simulink model "rr_arm_control"  (R2026a)
settings: Solver=VariableStepAuto  MaxStep=1E-03
InitFcn:
  | rr_arm_control_init;
values from neighbouring files (symbols this model uses):
  b1 = 0.9    [rr_arm_control_init.m]
  b2 = 0.9    [rr_arm_control_init.m]
  g = 9.81    [rr_arm_control_init.m]
  G1 = blkdiag(diag([Ixx1,Iyy1,Izz1]),m1*eye(3))    [rr_arm_control_init.m]
  G2 = blkdiag(diag([Ixx2,Iyy2,Izz2]),m2*eye(3))    [rr_arm_control_init.m]
  M1 = [ ... (first row only)    [rr_arm_control_init.m]
  M2 = [ ... (first row only)    [rr_arm_control_init.m]
  params = [Iyy1,Iyy2,m1,m2,l1,l2,b1,b2,g].'    [rr_arm_control_init.m]
  S1 = rscrew('y',[0,0,0])    [rr_arm_control_init.m]
  S2 = rscrew('y',[l1,0,0])    [rr_arm_control_init.m]
(part 2 of 2)

== system rr_arm_control/gravity_link_2/tform_adjoint/vec2skew ==
  x : Inport
  Constant : Constant  Value=0
  Demux : Demux  Outputs=3
  Gain : Gain  Gain=-1
  Gain1 : Gain  Gain=-1
  Gain2 : Gain  Gain=-1
  Matrix Concatenate : Concatenate  NumInputs=3  Mode=Multidimensional array  ConcatenateDimension=2
  Mux : Mux  Inputs=3
  Mux1 : Mux  Inputs=3
  Mux2 : Mux  Inputs=3
  "[x]" : Outport
  wires:
  Mux1/1 -> Matrix Concatenate/2
  Mux/1 -> Matrix Concatenate/1
  Mux2/1 -> Matrix Concatenate/3
  Matrix Concatenate/1 -> "[x]"/1
  Gain/1 -> Mux/3
  Gain1/1 -> Mux1/1
  Gain2/1 -> Mux2/2
  Constant/1 -> Mux/1, Mux1/2, Mux2/3
  x/1 -> Demux/1
  Demux/3 -> Gain1/1, Mux/2  "z"
  Demux/2 -> Mux2/1, Gain/1  "y"
  Demux/1 -> Gain2/1, Mux1/3  "x"

== system rr_arm_control/link_1/productOfExponentials/Subsystem1 ==
  S : Inport
  q : Inport  Port=2
  Reshape : Reshape  OutputDimensionality=Column vector (2-D)
  Selector : Selector  InputPortWidth=6  IndexOptions=Index vector (dialog)  Indices=1:3  OutputSizes=1
  axisAngleToRotMat : Subsystem
  screwDistanceToPos : Subsystem
  tform : Subsystem
  T : Outport
  wires:
  S/1 -> Reshape/1
  Selector/1 -> axisAngleToRotMat/1(w)  "w"
  q/1 -> screwDistanceToPos/2(q), axisAngleToRotMat/2(q)
  axisAngleToRotMat/1(R) -> tform/1(R)
  tform/1(T) -> T/1
  screwDistanceToPos/1(p) -> tform/2(p)
  Reshape/1 -> screwDistanceToPos/1(S), Selector/1

== system rr_arm_control/link_1/spaceJacobian/angle_screw_to_tform ==
  S : Inport
  q : Inport  Port=2
  Reshape : Reshape  OutputDimensionality=Column vector (2-D)
  Selector : Selector  InputPortWidth=6  IndexOptions=Index vector (dialog)  Indices=1:3  OutputSizes=1
  axisAngleToRotMat : Subsystem
  screwDistanceToPos : Subsystem
  tform : Subsystem
  T : Outport
  wires:
  S/1 -> Reshape/1
  Selector/1 -> axisAngleToRotMat/1(w)  "w"
  q/1 -> screwDistanceToPos/2(q), axisAngleToRotMat/2(q)
  axisAngleToRotMat/1(R) -> tform/1(R)
  tform/1(T) -> T/1
  screwDistanceToPos/1(p) -> tform/2(p)
  Reshape/1 -> screwDistanceToPos/1(S), Selector/1

== system rr_arm_control/link_1/spaceJacobian/tform_adjoint ==
  T : Inport
  Constant : Constant  Value=zeros(3)
  Matrix Concatenate : Concatenate  Mode=Multidimensional array  ConcatenateDimension=2
  Matrix Concatenate1 : Concatenate  Mode=Multidimensional array  ConcatenateDimension=2
  Matrix Concatenate2 : Concatenate  Mode=Multidimensional array
  Matrix Multiply : Product  Multiplication=Matrix(*)
  Selector : Selector  NumberOfDimensions=2  InputPortWidth=3  IndexOptions=Index vector (dialog),Index vector (dialog)  Indices=1:3,1:3  OutputSizes=1,1
  Selector1 : Selector  NumberOfDimensions=2  InputPortWidth=3  IndexOptions=Index vector (dialog),Index vector (dialog)  Indices=1:3,4  OutputSizes=1,1
  vec2skew : Subsystem
  Ad : Outport
  wires:
  Selector1/1 -> vec2skew/1(x)
  Selector/1 -> Matrix Multiply/2, Matrix Concatenate1/2, Matrix Concatenate/1
  Constant/1 -> Matrix Concatenate/2
  vec2skew/1("[x]") -> Matrix Multiply/1
  Matrix Multiply/1 -> Matrix Concatenate1/1
  Matrix Concatenate1/1 -> Matrix Concatenate2/2
  Matrix Concatenate/1 -> Matrix Concatenate2/1
  Matrix Concatenate2/1 -> Ad/1
  T/1 -> Selector1/1, Selector/1

== system rr_arm_control/link_1/spaceJacobianRate/angle_screw_to_tform ==
  S : Inport
  q : Inport  Port=2
  Reshape : Reshape  OutputDimensionality=Column vector (2-D)
  Selector : Selector  InputPortWidth=6  IndexOptions=Index vector (dialog)  Indices=1:3  OutputSizes=1
  axisAngleToRotMat : Subsystem
  screwDistanceToPos : Subsystem
  tform : Subsystem
  T : Outport
  wires:
  S/1 -> Reshape/1
  Selector/1 -> axisAngleToRotMat/1(w)  "w"
  q/1 -> screwDistanceToPos/2(q), axisAngleToRotMat/2(q)
  axisAngleToRotMat/1(R) -> tform/1(R)
  tform/1(T) -> T/1
  screwDistanceToPos/1(p) -> tform/2(p)
  Reshape/1 -> screwDistanceToPos/1(S), Selector/1

== system rr_arm_control/link_1/spaceJacobianRate/tform_adjoint ==
  T : Inport
  Constant : Constant  Value=zeros(3)
  Matrix Concatenate : Concatenate  Mode=Multidimensional array  ConcatenateDimension=2
  Matrix Concatenate1 : Concatenate  Mode=Multidimensional array  ConcatenateDimension=2
  Matrix Concatenate2 : Concatenate  Mode=Multidimensional array
  Matrix Multiply : Product  Multiplication=Matrix(*)
  Selector : Selector  NumberOfDimensions=2  InputPortWidth=3  IndexOptions=Index vector (dialog),Index vector (dialog)  Indices=1:3,1:3  OutputSizes=1,1
  Selector1 : Selector  NumberOfDimensions=2  InputPortWidth=3  IndexOptions=Index vector (dialog),Index vector (dialog)  Indices=1:3,4  OutputSizes=1,1
  vec2skew : Subsystem
  Ad : Outport
  wires:
  Selector1/1 -> vec2skew/1(x)
  Selector/1 -> Matrix Multiply/2, Matrix Concatenate1/2, Matrix Concatenate/1
  Constant/1 -> Matrix Concatenate/2
  vec2skew/1("[x]") -> Matrix Multiply/1
  Matrix Multiply/1 -> Matrix Concatenate1/1
  Matrix Concatenate1/1 -> Matrix Concatenate2/2
  Matrix Concatenate/1 -> Matrix Concatenate2/1
  Matrix Concatenate2/1 -> Ad/1
  T/1 -> Selector1/1, Selector/1

== system rr_arm_control/link_1/spaceJacobianRate/twist_adjoint ==
  V : Inport
  Constant : Constant  Value=zeros(3)
  Matrix Concatenate : Concatenate  Mode=Multidimensional array  ConcatenateDimension=2
  Matrix Concatenate1 : Concatenate  Mode=Multidimensional array  ConcatenateDimension=2
  Matrix Concatenate2 : Concatenate  Mode=Multidimensional array
  Selector : Selector  InputPortWidth=6  IndexOptions=Index vector (dialog)  Indices=1:3  OutputSizes=1
  Selector1 : Selector  InputPortWidth=6  IndexOptions=Index vector (dialog)  Indices=4:6  OutputSizes=1
  "[v]" : Subsystem
  "[w]" : Subsystem
  adV : Outport
  wires:
  Selector/1 -> "[w]"/1(x)
  Constant/1 -> Matrix Concatenate/2
  Matrix Concatenate1/1 -> Matrix Concatenate2/2
  Matrix Concatenate/1 -> Matrix Concatenate2/1
  Matrix Concatenate2/1 -> adV/1
  V/1 -> Selector1/1, Selector/1
  "[w]"/1("[x]") -> Matrix Concatenate1/2, Matrix Concatenate/1
  Selector1/1 -> "[v]"/1(x)
  "[v]"/1("[x]") -> Matrix Concatenate1/1

== system rr_arm_control/link_1/tform_adjoint/vec2skew ==
  x : Inport
  Constant : Constant  Value=0
  Demux : Demux  Outputs=3
  Gain : Gain  Gain=-1
  Gain1 : Gain  Gain=-1
  Gain2 : Gain  Gain=-1
  Matrix Concatenate : Concatenate  NumInputs=3  Mode=Multidimensional array  ConcatenateDimension=2
  Mux : Mux  Inputs=3
  Mux1 : Mux  Inputs=3
  Mux2 : Mux  Inputs=3
  "[x]" : Outport
  wires:
  Mux1/1 -> Matrix Concatenate/2
  Mux/1 -> Matrix Concatenate/1
  Mux2/1 -> Matrix Concatenate/3
  Matrix Concatenate/1 -> "[x]"/1
  Gain/1 -> Mux/3
  Gain1/1 -> Mux1/1
  Gain2/1 -> Mux2/2
  Constant/1 -> Mux/1, Mux1/2, Mux2/3
  x/1 -> Demux/1
  Demux/3 -> Gain1/1, Mux/2  "z"
  Demux/2 -> Mux2/1, Gain/1  "y"
  Demux/1 -> Gain2/1, Mux1/3  "x"

== system rr_arm_control/link_1/twist_adjoint/[v] ==
  x : Inport
  Constant : Constant  Value=0
  Demux : Demux  Outputs=3
  Gain : Gain  Gain=-1
  Gain1 : Gain  Gain=-1
  Gain2 : Gain  Gain=-1
  Matrix Concatenate : Concatenate  NumInputs=3  Mode=Multidimensional array  ConcatenateDimension=2
  Mux : Mux  Inputs=3
  Mux1 : Mux  Inputs=3
  Mux2 : Mux  Inputs=3
  "[x]" : Outport
  wires:
  Mux1/1 -> Matrix Concatenate/2
  Mux/1 -> Matrix Concatenate/1
  Mux2/1 -> Matrix Concatenate/3
  Matrix Concatenate/1 -> "[x]"/1
  Gain/1 -> Mux/3
  Gain1/1 -> Mux1/1
  Gain2/1 -> Mux2/2
  Constant/1 -> Mux/1, Mux1/2, Mux2/3
  x/1 -> Demux/1
  Demux/3 -> Gain1/1, Mux/2  "z"
  Demux/2 -> Mux2/1, Gain/1  "y"
  Demux/1 -> Gain2/1, Mux1/3  "x"

== system rr_arm_control/link_1/twist_adjoint/[w] ==
  x : Inport
  Constant : Constant  Value=0
  Demux : Demux  Outputs=3
  Gain : Gain  Gain=-1
  Gain1 : Gain  Gain=-1
  Gain2 : Gain  Gain=-1
  Matrix Concatenate : Concatenate  NumInputs=3  Mode=Multidimensional array  ConcatenateDimension=2
  Mux : Mux  Inputs=3
  Mux1 : Mux  Inputs=3
  Mux2 : Mux  Inputs=3
  "[x]" : Outport
  wires:
  Mux1/1 -> Matrix Concatenate/2
  Mux/1 -> Matrix Concatenate/1
  Mux2/1 -> Matrix Concatenate/3
  Matrix Concatenate/1 -> "[x]"/1
  Gain/1 -> Mux/3
  Gain1/1 -> Mux1/1
  Gain2/1 -> Mux2/2
  Constant/1 -> Mux/1, Mux1/2, Mux2/3
  x/1 -> Demux/1
  Demux/3 -> Gain1/1, Mux/2  "z"
  Demux/2 -> Mux2/1, Gain/1  "y"
  Demux/1 -> Gain2/1, Mux1/3  "x"

== system rr_arm_control/link_2/productOfExponentials/Subsystem1 ==
  S : Inport
  q : Inport  Port=2
  Reshape : Reshape  OutputDimensionality=Column vector (2-D)
  Selector : Selector  InputPortWidth=6  IndexOptions=Index vector (dialog)  Indices=1:3  OutputSizes=1
  axisAngleToRotMat : Subsystem
  screwDistanceToPos : Subsystem
  tform : Subsystem
  T : Outport
  wires:
  S/1 -> Reshape/1
  Selector/1 -> axisAngleToRotMat/1(w)  "w"
  q/1 -> screwDistanceToPos/2(q), axisAngleToRotMat/2(q)
  axisAngleToRotMat/1(R) -> tform/1(R)
  tform/1(T) -> T/1
  screwDistanceToPos/1(p) -> tform/2(p)
  Reshape/1 -> screwDistanceToPos/1(S), Selector/1

== system rr_arm_control/link_2/spaceJacobian/angle_screw_to_tform ==
  S : Inport
  q : Inport  Port=2
  Reshape : Reshape  OutputDimensionality=Column vector (2-D)
  Selector : Selector  InputPortWidth=6  IndexOptions=Index vector (dialog)  Indices=1:3  OutputSizes=1
  axisAngleToRotMat : Subsystem
  screwDistanceToPos : Subsystem
  tform : Subsystem
  T : Outport
  wires:
  S/1 -> Reshape/1
  Selector/1 -> axisAngleToRotMat/1(w)  "w"
  q/1 -> screwDistanceToPos/2(q), axisAngleToRotMat/2(q)
  axisAngleToRotMat/1(R) -> tform/1(R)
  tform/1(T) -> T/1
  screwDistanceToPos/1(p) -> tform/2(p)
  Reshape/1 -> screwDistanceToPos/1(S), Selector/1

== system rr_arm_control/link_2/spaceJacobian/tform_adjoint ==
  T : Inport
  Constant : Constant  Value=zeros(3)
  Matrix Concatenate : Concatenate  Mode=Multidimensional array  ConcatenateDimension=2
  Matrix Concatenate1 : Concatenate  Mode=Multidimensional array  ConcatenateDimension=2
  Matrix Concatenate2 : Concatenate  Mode=Multidimensional array
  Matrix Multiply : Product  Multiplication=Matrix(*)
  Selector : Selector  NumberOfDimensions=2  InputPortWidth=3  IndexOptions=Index vector (dialog),Index vector (dialog)  Indices=1:3,1:3  OutputSizes=1,1
  Selector1 : Selector  NumberOfDimensions=2  InputPortWidth=3  IndexOptions=Index vector (dialog),Index vector (dialog)  Indices=1:3,4  OutputSizes=1,1
  vec2skew : Subsystem
  Ad : Outport
  wires:
  Selector1/1 -> vec2skew/1(x)
  Selector/1 -> Matrix Multiply/2, Matrix Concatenate1/2, Matrix Concatenate/1
  Constant/1 -> Matrix Concatenate/2
  vec2skew/1("[x]") -> Matrix Multiply/1
  Matrix Multiply/1 -> Matrix Concatenate1/1
  Matrix Concatenate1/1 -> Matrix Concatenate2/2
  Matrix Concatenate/1 -> Matrix Concatenate2/1
  Matrix Concatenate2/1 -> Ad/1
  T/1 -> Selector1/1, Selector/1

== system rr_arm_control/link_2/spaceJacobianRate/angle_screw_to_tform ==
  S : Inport
  q : Inport  Port=2
  Reshape : Reshape  OutputDimensionality=Column vector (2-D)
  Selector : Selector  InputPortWidth=6  IndexOptions=Index vector (dialog)  Indices=1:3  OutputSizes=1
  axisAngleToRotMat : Subsystem
  screwDistanceToPos : Subsystem
  tform : Subsystem
  T : Outport
  wires:
  S/1 -> Reshape/1
  Selector/1 -> axisAngleToRotMat/1(w)  "w"
  q/1 -> screwDistanceToPos/2(q), axisAngleToRotMat/2(q)
  axisAngleToRotMat/1(R) -> tform/1(R)
  tform/1(T) -> T/1
  screwDistanceToPos/1(p) -> tform/2(p)
  Reshape/1 -> screwDistanceToPos/1(S), Selector/1

== system rr_arm_control/link_2/spaceJacobianRate/tform_adjoint ==
  T : Inport
  Constant : Constant  Value=zeros(3)
  Matrix Concatenate : Concatenate  Mode=Multidimensional array  ConcatenateDimension=2
  Matrix Concatenate1 : Concatenate  Mode=Multidimensional array  ConcatenateDimension=2
  Matrix Concatenate2 : Concatenate  Mode=Multidimensional array
  Matrix Multiply : Product  Multiplication=Matrix(*)
  Selector : Selector  NumberOfDimensions=2  InputPortWidth=3  IndexOptions=Index vector (dialog),Index vector (dialog)  Indices=1:3,1:3  OutputSizes=1,1
  Selector1 : Selector  NumberOfDimensions=2  InputPortWidth=3  IndexOptions=Index vector (dialog),Index vector (dialog)  Indices=1:3,4  OutputSizes=1,1
  vec2skew : Subsystem
  Ad : Outport
  wires:
  Selector1/1 -> vec2skew/1(x)
  Selector/1 -> Matrix Multiply/2, Matrix Concatenate1/2, Matrix Concatenate/1
  Constant/1 -> Matrix Concatenate/2
  vec2skew/1("[x]") -> Matrix Multiply/1
  Matrix Multiply/1 -> Matrix Concatenate1/1
  Matrix Concatenate1/1 -> Matrix Concatenate2/2
  Matrix Concatenate/1 -> Matrix Concatenate2/1
  Matrix Concatenate2/1 -> Ad/1
  T/1 -> Selector1/1, Selector/1

== system rr_arm_control/link_2/spaceJacobianRate/twist_adjoint ==
  V : Inport
  Constant : Constant  Value=zeros(3)
  Matrix Concatenate : Concatenate  Mode=Multidimensional array  ConcatenateDimension=2
  Matrix Concatenate1 : Concatenate  Mode=Multidimensional array  ConcatenateDimension=2
  Matrix Concatenate2 : Concatenate  Mode=Multidimensional array
  Selector : Selector  InputPortWidth=6  IndexOptions=Index vector (dialog)  Indices=1:3  OutputSizes=1
  Selector1 : Selector  InputPortWidth=6  IndexOptions=Index vector (dialog)  Indices=4:6  OutputSizes=1
  "[v]" : Subsystem
  "[w]" : Subsystem
  adV : Outport
  wires:
  Selector/1 -> "[w]"/1(x)
  Constant/1 -> Matrix Concatenate/2
  Matrix Concatenate1/1 -> Matrix Concatenate2/2
  Matrix Concatenate/1 -> Matrix Concatenate2/1
  Matrix Concatenate2/1 -> adV/1
  V/1 -> Selector1/1, Selector/1
  "[w]"/1("[x]") -> Matrix Concatenate1/2, Matrix Concatenate/1
  Selector1/1 -> "[v]"/1(x)
  "[v]"/1("[x]") -> Matrix Concatenate1/1

== system rr_arm_control/link_2/tform_adjoint/vec2skew ==
  x : Inport
  Constant : Constant  Value=0
  Demux : Demux  Outputs=3
  Gain : Gain  Gain=-1
  Gain1 : Gain  Gain=-1
  Gain2 : Gain  Gain=-1
  Matrix Concatenate : Concatenate  NumInputs=3  Mode=Multidimensional array  ConcatenateDimension=2
  Mux : Mux  Inputs=3
  Mux1 : Mux  Inputs=3
  Mux2 : Mux  Inputs=3
  "[x]" : Outport
  wires:
  Mux1/1 -> Matrix Concatenate/2
  Mux/1 -> Matrix Concatenate/1
  Mux2/1 -> Matrix Concatenate/3
  Matrix Concatenate/1 -> "[x]"/1
  Gain/1 -> Mux/3
  Gain1/1 -> Mux1/1
  Gain2/1 -> Mux2/2
  Constant/1 -> Mux/1, Mux1/2, Mux2/3
  x/1 -> Demux/1
  Demux/3 -> Gain1/1, Mux/2  "z"
  Demux/2 -> Mux2/1, Gain/1  "y"
  Demux/1 -> Gain2/1, Mux1/3  "x"

== system rr_arm_control/link_2/twist_adjoint/[v] ==
  x : Inport
  Constant : Constant  Value=0
  Demux : Demux  Outputs=3
  Gain : Gain  Gain=-1
  Gain1 : Gain  Gain=-1
  Gain2 : Gain  Gain=-1
  Matrix Concatenate : Concatenate  NumInputs=3  Mode=Multidimensional array  ConcatenateDimension=2
  Mux : Mux  Inputs=3
  Mux1 : Mux  Inputs=3
  Mux2 : Mux  Inputs=3
  "[x]" : Outport
  wires:
  Mux1/1 -> Matrix Concatenate/2
  Mux/1 -> Matrix Concatenate/1
  Mux2/1 -> Matrix Concatenate/3
  Matrix Concatenate/1 -> "[x]"/1
  Gain/1 -> Mux/3
  Gain1/1 -> Mux1/1
  Gain2/1 -> Mux2/2
  Constant/1 -> Mux/1, Mux1/2, Mux2/3
  x/1 -> Demux/1
  Demux/3 -> Gain1/1, Mux/2  "z"
  Demux/2 -> Mux2/1, Gain/1  "y"
  Demux/1 -> Gain2/1, Mux1/3  "x"

== system rr_arm_control/link_2/twist_adjoint/[w] ==
  x : Inport
  Constant : Constant  Value=0
  Demux : Demux  Outputs=3
  Gain : Gain  Gain=-1
  Gain1 : Gain  Gain=-1
  Gain2 : Gain  Gain=-1
  Matrix Concatenate : Concatenate  NumInputs=3  Mode=Multidimensional array  ConcatenateDimension=2
  Mux : Mux  Inputs=3
  Mux1 : Mux  Inputs=3
  Mux2 : Mux  Inputs=3
  "[x]" : Outport
  wires:
  Mux1/1 -> Matrix Concatenate/2
  Mux/1 -> Matrix Concatenate/1
  Mux2/1 -> Matrix Concatenate/3
  Matrix Concatenate/1 -> "[x]"/1
  Gain/1 -> Mux/3
  Gain1/1 -> Mux1/1
  Gain2/1 -> Mux2/2
  Constant/1 -> Mux/1, Mux1/2, Mux2/3
  x/1 -> Demux/1
  Demux/3 -> Gain1/1, Mux/2  "z"
  Demux/2 -> Mux2/1, Gain/1  "y"
  Demux/1 -> Gain2/1, Mux1/3  "x"

== system rr_arm_control/link_1/productOfExponentials/Subsystem1/axisAngleToRotMat ==
  w : Inport
  q : Inport  Port=2
  Constant : Constant
  Cos : Trigonometry  Operator=cos
  I : Constant  Value=eye(3)
  Matrix Multiply : Product  Multiplication=Matrix(*)
  Product : Product
  Product1 : Product
  Sin : Trigonometry
  Sum : Sum  Inputs=|+-
  Sum1 : Sum  Inputs=|++
  Sum2 : Sum  Inputs=|++
  vec2skew : Subsystem
  R : Outport
  wires:
  Cos/1 -> Sum/2
  Sum1/1 -> Sum2/1
  Sum/1 -> Product1/2
  Matrix Multiply/1 -> Product1/1  "[w]^2"
  Product1/1 -> Sum1/2
  Constant/1 -> Sum/1
  Product/1 -> Sum1/1
  I/1 -> Sum2/2
  vec2skew/1("[x]") -> Matrix Multiply/2, Matrix Multiply/1, Product/1  "[w]"
  Sin/1 -> Product/2
  q/1 -> Cos/1, Sin/1
  Sum2/1 -> R/1
  w/1 -> vec2skew/1(x)

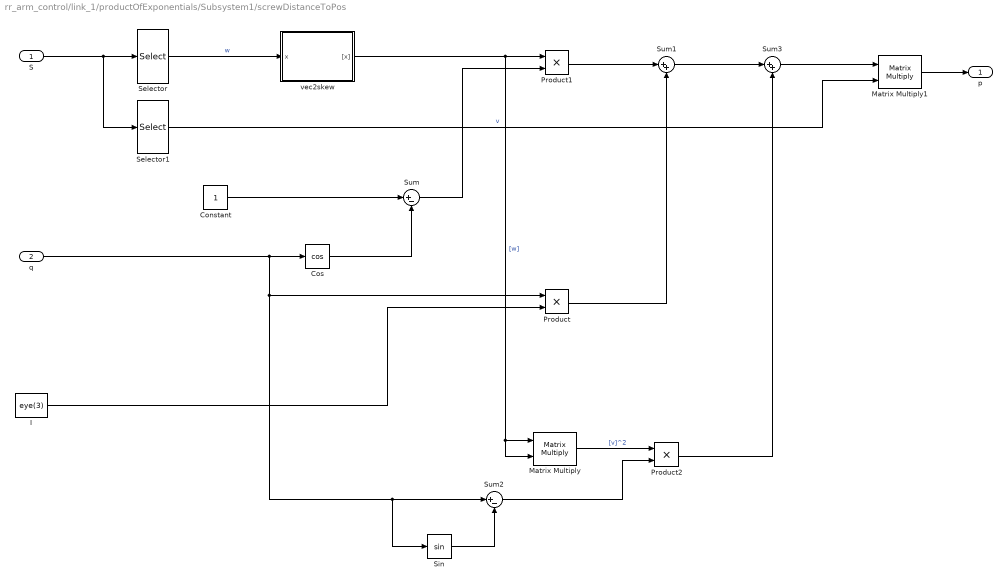
== system rr_arm_control/link_1/productOfExponentials/Subsystem1/screwDistanceToPos ==
  S : Inport
  q : Inport  Port=2
  Constant : Constant
  Cos : Trigonometry  Operator=cos
  I : Constant  Value=eye(3)
  Matrix Multiply : Product  Multiplication=Matrix(*)
  Matrix Multiply1 : Product  Multiplication=Matrix(*)
  Product : Product
  Product1 : Product
  Product2 : Product
  Selector : Selector  InputPortWidth=6  IndexOptions=Index vector (dialog)  Indices=1:3  OutputSizes=1
  Selector1 : Selector  InputPortWidth=6  IndexOptions=Index vector (dialog)  Indices=4:6  OutputSizes=1
  Sin : Trigonometry
  Sum : Sum  Inputs=|+-
  Sum1 : Sum  Inputs=|++
  Sum2 : Sum  Inputs=|+-
  Sum3 : Sum  Inputs=|++
  vec2skew : Subsystem
  p : Outport
  wires:
  Product/1 -> Sum1/2
  q/1 -> Cos/1, Product/1, Sin/1, Sum2/1
  Cos/1 -> Sum/2
  Constant/1 -> Sum/1
  vec2skew/1("[x]") -> Matrix Multiply/2, Matrix Multiply/1, Product1/1  "[w]"
  Sum2/1 -> Product2/2
  I/1 -> Product/2
  Product1/1 -> Sum1/1
  Sum/1 -> Product1/2
  Matrix Multiply/1 -> Product2/1  "[v]^2"
  Sum3/1 -> Matrix Multiply1/1
  Product2/1 -> Sum3/2
  Sin/1 -> Sum2/2
  Sum1/1 -> Sum3/1
  Selector1/1 -> Matrix Multiply1/2  "v"
  Matrix Multiply1/1 -> p/1
  Selector/1 -> vec2skew/1(x)  "w"
  S/1 -> Selector1/1, Selector/1

== system rr_arm_control/link_1/productOfExponentials/Subsystem1/tform ==
  R : Inport
  p : Inport  Port=2
  Constant : Constant  Value=[0,0,0,1]
  Matrix Concatenate : Concatenate  Mode=Multidimensional array  ConcatenateDimension=2
  Matrix Concatenate2 : Concatenate  Mode=Multidimensional array
  Reshape : Reshape  OutputDimensionality=Row vector (2-D)
  T : Outport
  wires:
  p/1 -> Matrix Concatenate/2
  Constant/1 -> Reshape/1
  Matrix Concatenate/1 -> Matrix Concatenate2/1
  Matrix Concatenate2/1 -> T/1
  R/1 -> Matrix Concatenate/1
  Reshape/1 -> Matrix Concatenate2/2

== system rr_arm_control/link_1/spaceJacobian/angle_screw_to_tform/axisAngleToRotMat ==
  w : Inport
  q : Inport  Port=2
  Constant : Constant
  Cos : Trigonometry  Operator=cos
  I : Constant  Value=eye(3)
  Matrix Multiply : Product  Multiplication=Matrix(*)
  Product : Product
  Product1 : Product
  Sin : Trigonometry
  Sum : Sum  Inputs=|+-
  Sum1 : Sum  Inputs=|++
  Sum2 : Sum  Inputs=|++
  vec2skew : Subsystem
  R : Outport
  wires:
  Cos/1 -> Sum/2
  Sum1/1 -> Sum2/1
  Sum/1 -> Product1/2
  Matrix Multiply/1 -> Product1/1  "[w]^2"
  Product1/1 -> Sum1/2
  Constant/1 -> Sum/1
  Product/1 -> Sum1/1
  I/1 -> Sum2/2
  vec2skew/1("[x]") -> Matrix Multiply/2, Matrix Multiply/1, Product/1  "[w]"
  Sin/1 -> Product/2
  q/1 -> Cos/1, Sin/1
  Sum2/1 -> R/1
  w/1 -> vec2skew/1(x)

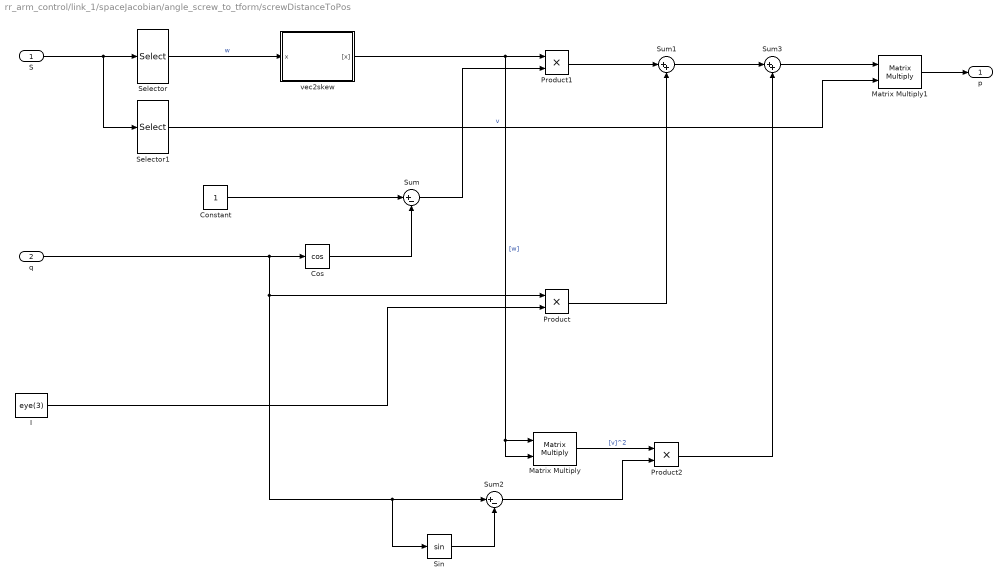
== system rr_arm_control/link_1/spaceJacobian/angle_screw_to_tform/screwDistanceToPos ==
  S : Inport
  q : Inport  Port=2
  Constant : Constant
  Cos : Trigonometry  Operator=cos
  I : Constant  Value=eye(3)
  Matrix Multiply : Product  Multiplication=Matrix(*)
  Matrix Multiply1 : Product  Multiplication=Matrix(*)
  Product : Product
  Product1 : Product
  Product2 : Product
  Selector : Selector  InputPortWidth=6  IndexOptions=Index vector (dialog)  Indices=1:3  OutputSizes=1
  Selector1 : Selector  InputPortWidth=6  IndexOptions=Index vector (dialog)  Indices=4:6  OutputSizes=1
  Sin : Trigonometry
  Sum : Sum  Inputs=|+-
  Sum1 : Sum  Inputs=|++
  Sum2 : Sum  Inputs=|+-
  Sum3 : Sum  Inputs=|++
  vec2skew : Subsystem
  p : Outport
  wires:
  Product/1 -> Sum1/2
  q/1 -> Cos/1, Product/1, Sin/1, Sum2/1
  Cos/1 -> Sum/2
  Constant/1 -> Sum/1
  vec2skew/1("[x]") -> Matrix Multiply/2, Matrix Multiply/1, Product1/1  "[w]"
  Sum2/1 -> Product2/2
  I/1 -> Product/2
  Product1/1 -> Sum1/1
  Sum/1 -> Product1/2
  Matrix Multiply/1 -> Product2/1  "[v]^2"
  Sum3/1 -> Matrix Multiply1/1
  Product2/1 -> Sum3/2
  Sin/1 -> Sum2/2
  Sum1/1 -> Sum3/1
  Selector1/1 -> Matrix Multiply1/2  "v"
  Matrix Multiply1/1 -> p/1
  Selector/1 -> vec2skew/1(x)  "w"
  S/1 -> Selector1/1, Selector/1

== system rr_arm_control/link_1/spaceJacobian/angle_screw_to_tform/tform ==
  R : Inport
  p : Inport  Port=2
  Constant : Constant  Value=[0,0,0,1]
  Matrix Concatenate : Concatenate  Mode=Multidimensional array  ConcatenateDimension=2
  Matrix Concatenate2 : Concatenate  Mode=Multidimensional array
  Reshape : Reshape  OutputDimensionality=Row vector (2-D)
  T : Outport
  wires:
  p/1 -> Matrix Concatenate/2
  Constant/1 -> Reshape/1
  Matrix Concatenate/1 -> Matrix Concatenate2/1
  Matrix Concatenate2/1 -> T/1
  R/1 -> Matrix Concatenate/1
  Reshape/1 -> Matrix Concatenate2/2

== system rr_arm_control/link_1/spaceJacobian/tform_adjoint/vec2skew ==
  x : Inport
  Constant : Constant  Value=0
  Demux : Demux  Outputs=3
  Gain : Gain  Gain=-1
  Gain1 : Gain  Gain=-1
  Gain2 : Gain  Gain=-1
  Matrix Concatenate : Concatenate  NumInputs=3  Mode=Multidimensional array  ConcatenateDimension=2
  Mux : Mux  Inputs=3
  Mux1 : Mux  Inputs=3
  Mux2 : Mux  Inputs=3
  "[x]" : Outport
  wires:
  Mux1/1 -> Matrix Concatenate/2
  Mux/1 -> Matrix Concatenate/1
  Mux2/1 -> Matrix Concatenate/3
  Matrix Concatenate/1 -> "[x]"/1
  Gain/1 -> Mux/3
  Gain1/1 -> Mux1/1
  Gain2/1 -> Mux2/2
  Constant/1 -> Mux/1, Mux1/2, Mux2/3
  x/1 -> Demux/1
  Demux/3 -> Gain1/1, Mux/2  "z"
  Demux/2 -> Mux2/1, Gain/1  "y"
  Demux/1 -> Gain2/1, Mux1/3  "x"

== system rr_arm_control/link_1/spaceJacobianRate/angle_screw_to_tform/axisAngleToRotMat ==
  w : Inport
  q : Inport  Port=2
  Constant : Constant
  Cos : Trigonometry  Operator=cos
  I : Constant  Value=eye(3)
  Matrix Multiply : Product  Multiplication=Matrix(*)
  Product : Product
  Product1 : Product
  Sin : Trigonometry
  Sum : Sum  Inputs=|+-
  Sum1 : Sum  Inputs=|++
  Sum2 : Sum  Inputs=|++
  vec2skew : Subsystem
  R : Outport
  wires:
  Cos/1 -> Sum/2
  Sum1/1 -> Sum2/1
  Sum/1 -> Product1/2
  Matrix Multiply/1 -> Product1/1  "[w]^2"
  Product1/1 -> Sum1/2
  Constant/1 -> Sum/1
  Product/1 -> Sum1/1
  I/1 -> Sum2/2
  vec2skew/1("[x]") -> Matrix Multiply/2, Matrix Multiply/1, Product/1  "[w]"
  Sin/1 -> Product/2
  q/1 -> Cos/1, Sin/1
  Sum2/1 -> R/1
  w/1 -> vec2skew/1(x)

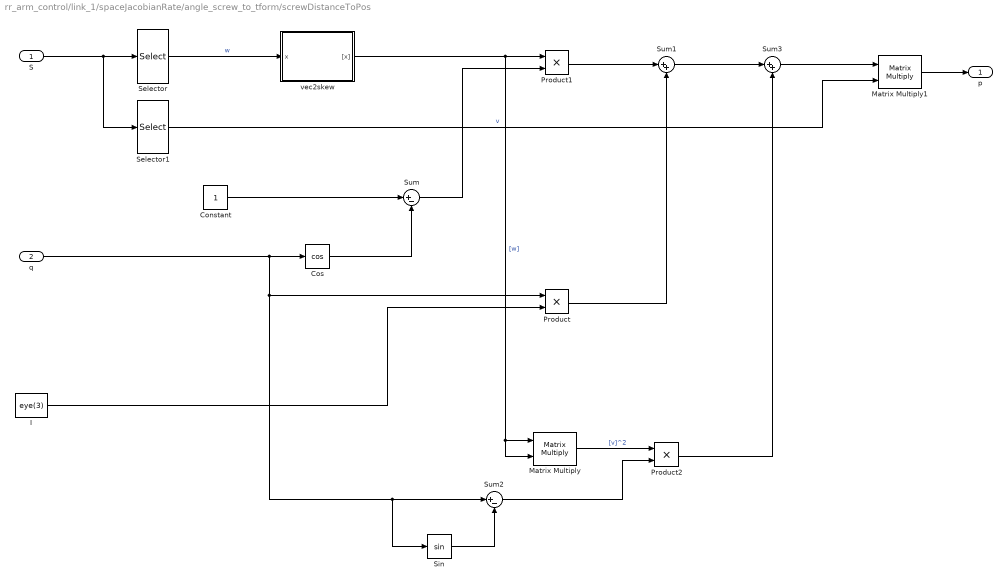
== system rr_arm_control/link_1/spaceJacobianRate/angle_screw_to_tform/screwDistanceToPos ==
  S : Inport
  q : Inport  Port=2
  Constant : Constant
  Cos : Trigonometry  Operator=cos
  I : Constant  Value=eye(3)
  Matrix Multiply : Product  Multiplication=Matrix(*)
  Matrix Multiply1 : Product  Multiplication=Matrix(*)
  Product : Product
  Product1 : Product
  Product2 : Product
  Selector : Selector  InputPortWidth=6  IndexOptions=Index vector (dialog)  Indices=1:3  OutputSizes=1
  Selector1 : Selector  InputPortWidth=6  IndexOptions=Index vector (dialog)  Indices=4:6  OutputSizes=1
  Sin : Trigonometry
  Sum : Sum  Inputs=|+-
  Sum1 : Sum  Inputs=|++
  Sum2 : Sum  Inputs=|+-
  Sum3 : Sum  Inputs=|++
  vec2skew : Subsystem
  p : Outport
  wires:
  Product/1 -> Sum1/2
  q/1 -> Cos/1, Product/1, Sin/1, Sum2/1
  Cos/1 -> Sum/2
  Constant/1 -> Sum/1
  vec2skew/1("[x]") -> Matrix Multiply/2, Matrix Multiply/1, Product1/1  "[w]"
  Sum2/1 -> Product2/2
  I/1 -> Product/2
  Product1/1 -> Sum1/1
  Sum/1 -> Product1/2
  Matrix Multiply/1 -> Product2/1  "[v]^2"
  Sum3/1 -> Matrix Multiply1/1
  Product2/1 -> Sum3/2
  Sin/1 -> Sum2/2
  Sum1/1 -> Sum3/1
  Selector1/1 -> Matrix Multiply1/2  "v"
  Matrix Multiply1/1 -> p/1
  Selector/1 -> vec2skew/1(x)  "w"
  S/1 -> Selector1/1, Selector/1

== system rr_arm_control/link_1/spaceJacobianRate/angle_screw_to_tform/tform ==
  R : Inport
  p : Inport  Port=2
  Constant : Constant  Value=[0,0,0,1]
  Matrix Concatenate : Concatenate  Mode=Multidimensional array  ConcatenateDimension=2
  Matrix Concatenate2 : Concatenate  Mode=Multidimensional array
  Reshape : Reshape  OutputDimensionality=Row vector (2-D)
  T : Outport
  wires:
  p/1 -> Matrix Concatenate/2
  Constant/1 -> Reshape/1
  Matrix Concatenate/1 -> Matrix Concatenate2/1
  Matrix Concatenate2/1 -> T/1
  R/1 -> Matrix Concatenate/1
  Reshape/1 -> Matrix Concatenate2/2

== system rr_arm_control/link_1/spaceJacobianRate/tform_adjoint/vec2skew ==
  x : Inport
  Constant : Constant  Value=0
  Demux : Demux  Outputs=3
  Gain : Gain  Gain=-1
  Gain1 : Gain  Gain=-1
  Gain2 : Gain  Gain=-1
  Matrix Concatenate : Concatenate  NumInputs=3  Mode=Multidimensional array  ConcatenateDimension=2
  Mux : Mux  Inputs=3
  Mux1 : Mux  Inputs=3
  Mux2 : Mux  Inputs=3
  "[x]" : Outport
  wires:
  Mux1/1 -> Matrix Concatenate/2
  Mux/1 -> Matrix Concatenate/1
  Mux2/1 -> Matrix Concatenate/3
  Matrix Concatenate/1 -> "[x]"/1
  Gain/1 -> Mux/3
  Gain1/1 -> Mux1/1
  Gain2/1 -> Mux2/2
  Constant/1 -> Mux/1, Mux1/2, Mux2/3
  x/1 -> Demux/1
  Demux/3 -> Gain1/1, Mux/2  "z"
  Demux/2 -> Mux2/1, Gain/1  "y"
  Demux/1 -> Gain2/1, Mux1/3  "x"

== system rr_arm_control/link_1/spaceJacobianRate/twist_adjoint/[v] ==
  x : Inport
  Constant : Constant  Value=0
  Demux : Demux  Outputs=3
  Gain : Gain  Gain=-1
  Gain1 : Gain  Gain=-1
  Gain2 : Gain  Gain=-1
  Matrix Concatenate : Concatenate  NumInputs=3  Mode=Multidimensional array  ConcatenateDimension=2
  Mux : Mux  Inputs=3
  Mux1 : Mux  Inputs=3
  Mux2 : Mux  Inputs=3
  "[x]" : Outport
  wires:
  Mux1/1 -> Matrix Concatenate/2
  Mux/1 -> Matrix Concatenate/1
  Mux2/1 -> Matrix Concatenate/3
  Matrix Concatenate/1 -> "[x]"/1
  Gain/1 -> Mux/3
  Gain1/1 -> Mux1/1
  Gain2/1 -> Mux2/2
  Constant/1 -> Mux/1, Mux1/2, Mux2/3
  x/1 -> Demux/1
  Demux/3 -> Gain1/1, Mux/2  "z"
  Demux/2 -> Mux2/1, Gain/1  "y"
  Demux/1 -> Gain2/1, Mux1/3  "x"

== system rr_arm_control/link_1/spaceJacobianRate/twist_adjoint/[w] ==
  x : Inport
  Constant : Constant  Value=0
  Demux : Demux  Outputs=3
  Gain : Gain  Gain=-1
  Gain1 : Gain  Gain=-1
  Gain2 : Gain  Gain=-1
  Matrix Concatenate : Concatenate  NumInputs=3  Mode=Multidimensional array  ConcatenateDimension=2
  Mux : Mux  Inputs=3
  Mux1 : Mux  Inputs=3
  Mux2 : Mux  Inputs=3
  "[x]" : Outport
  wires:
  Mux1/1 -> Matrix Concatenate/2
  Mux/1 -> Matrix Concatenate/1
  Mux2/1 -> Matrix Concatenate/3
  Matrix Concatenate/1 -> "[x]"/1
  Gain/1 -> Mux/3
  Gain1/1 -> Mux1/1
  Gain2/1 -> Mux2/2
  Constant/1 -> Mux/1, Mux1/2, Mux2/3
  x/1 -> Demux/1
  Demux/3 -> Gain1/1, Mux/2  "z"
  Demux/2 -> Mux2/1, Gain/1  "y"
  Demux/1 -> Gain2/1, Mux1/3  "x"

== system rr_arm_control/link_2/productOfExponentials/Subsystem1/axisAngleToRotMat ==
  w : Inport
  q : Inport  Port=2
  Constant : Constant
  Cos : Trigonometry  Operator=cos
  I : Constant  Value=eye(3)
  Matrix Multiply : Product  Multiplication=Matrix(*)
  Product : Product
  Product1 : Product
  Sin : Trigonometry
  Sum : Sum  Inputs=|+-
  Sum1 : Sum  Inputs=|++
  Sum2 : Sum  Inputs=|++
  vec2skew : Subsystem
  R : Outport
  wires:
  Cos/1 -> Sum/2
  Sum1/1 -> Sum2/1
  Sum/1 -> Product1/2
  Matrix Multiply/1 -> Product1/1  "[w]^2"
  Product1/1 -> Sum1/2
  Constant/1 -> Sum/1
  Product/1 -> Sum1/1
  I/1 -> Sum2/2
  vec2skew/1("[x]") -> Matrix Multiply/2, Matrix Multiply/1, Product/1  "[w]"
  Sin/1 -> Product/2
  q/1 -> Cos/1, Sin/1
  Sum2/1 -> R/1
  w/1 -> vec2skew/1(x)

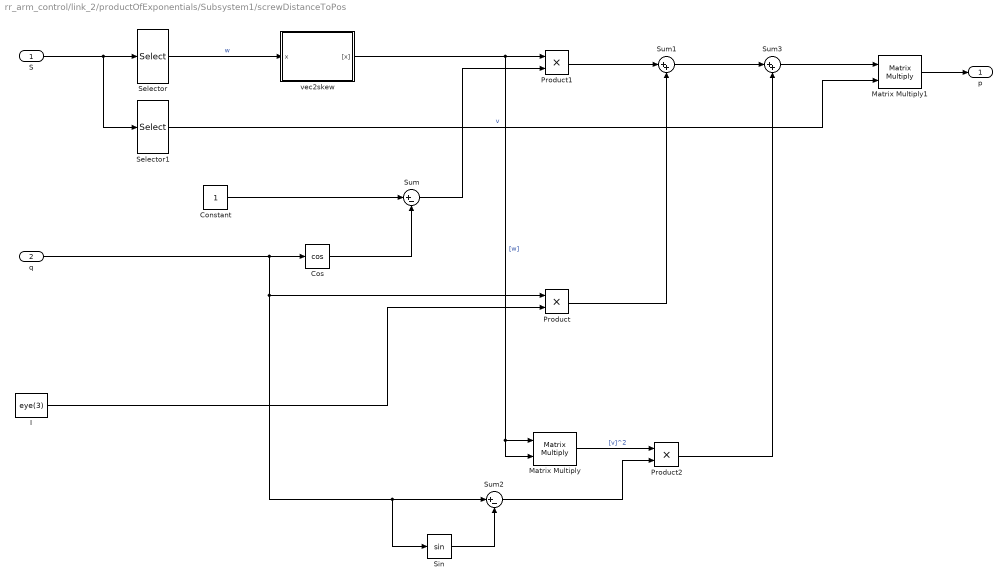
== system rr_arm_control/link_2/productOfExponentials/Subsystem1/screwDistanceToPos ==
  S : Inport
  q : Inport  Port=2
  Constant : Constant
  Cos : Trigonometry  Operator=cos
  I : Constant  Value=eye(3)
  Matrix Multiply : Product  Multiplication=Matrix(*)
  Matrix Multiply1 : Product  Multiplication=Matrix(*)
  Product : Product
  Product1 : Product
  Product2 : Product
  Selector : Selector  InputPortWidth=6  IndexOptions=Index vector (dialog)  Indices=1:3  OutputSizes=1
  Selector1 : Selector  InputPortWidth=6  IndexOptions=Index vector (dialog)  Indices=4:6  OutputSizes=1
  Sin : Trigonometry
  Sum : Sum  Inputs=|+-
  Sum1 : Sum  Inputs=|++
  Sum2 : Sum  Inputs=|+-
  Sum3 : Sum  Inputs=|++
  vec2skew : Subsystem
  p : Outport
  wires:
  Product/1 -> Sum1/2
  q/1 -> Cos/1, Product/1, Sin/1, Sum2/1
  Cos/1 -> Sum/2
  Constant/1 -> Sum/1
  vec2skew/1("[x]") -> Matrix Multiply/2, Matrix Multiply/1, Product1/1  "[w]"
  Sum2/1 -> Product2/2
  I/1 -> Product/2
  Product1/1 -> Sum1/1
  Sum/1 -> Product1/2
  Matrix Multiply/1 -> Product2/1  "[v]^2"
  Sum3/1 -> Matrix Multiply1/1
  Product2/1 -> Sum3/2
  Sin/1 -> Sum2/2
  Sum1/1 -> Sum3/1
  Selector1/1 -> Matrix Multiply1/2  "v"
  Matrix Multiply1/1 -> p/1
  Selector/1 -> vec2skew/1(x)  "w"
  S/1 -> Selector1/1, Selector/1

== system rr_arm_control/link_2/productOfExponentials/Subsystem1/tform ==
  R : Inport
  p : Inport  Port=2
  Constant : Constant  Value=[0,0,0,1]
  Matrix Concatenate : Concatenate  Mode=Multidimensional array  ConcatenateDimension=2
  Matrix Concatenate2 : Concatenate  Mode=Multidimensional array
  Reshape : Reshape  OutputDimensionality=Row vector (2-D)
  T : Outport
  wires:
  p/1 -> Matrix Concatenate/2
  Constant/1 -> Reshape/1
  Matrix Concatenate/1 -> Matrix Concatenate2/1
  Matrix Concatenate2/1 -> T/1
  R/1 -> Matrix Concatenate/1
  Reshape/1 -> Matrix Concatenate2/2

== system rr_arm_control/link_2/spaceJacobian/angle_screw_to_tform/axisAngleToRotMat ==
  w : Inport
  q : Inport  Port=2
  Constant : Constant
  Cos : Trigonometry  Operator=cos
  I : Constant  Value=eye(3)
  Matrix Multiply : Product  Multiplication=Matrix(*)
  Product : Product
  Product1 : Product
  Sin : Trigonometry
  Sum : Sum  Inputs=|+-
  Sum1 : Sum  Inputs=|++
  Sum2 : Sum  Inputs=|++
  vec2skew : Subsystem
  R : Outport
  wires:
  Cos/1 -> Sum/2
  Sum1/1 -> Sum2/1
  Sum/1 -> Product1/2
  Matrix Multiply/1 -> Product1/1  "[w]^2"
  Product1/1 -> Sum1/2
  Constant/1 -> Sum/1
  Product/1 -> Sum1/1
  I/1 -> Sum2/2
  vec2skew/1("[x]") -> Matrix Multiply/2, Matrix Multiply/1, Product/1  "[w]"
  Sin/1 -> Product/2
  q/1 -> Cos/1, Sin/1
  Sum2/1 -> R/1
  w/1 -> vec2skew/1(x)

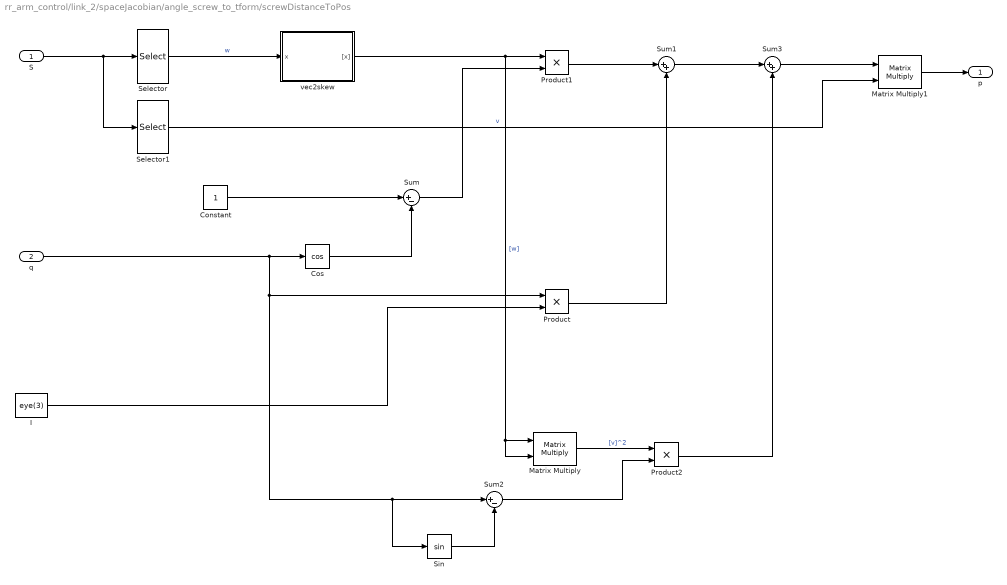
== system rr_arm_control/link_2/spaceJacobian/angle_screw_to_tform/screwDistanceToPos ==
  S : Inport
  q : Inport  Port=2
  Constant : Constant
  Cos : Trigonometry  Operator=cos
  I : Constant  Value=eye(3)
  Matrix Multiply : Product  Multiplication=Matrix(*)
  Matrix Multiply1 : Product  Multiplication=Matrix(*)
  Product : Product
  Product1 : Product
  Product2 : Product
  Selector : Selector  InputPortWidth=6  IndexOptions=Index vector (dialog)  Indices=1:3  OutputSizes=1
  Selector1 : Selector  InputPortWidth=6  IndexOptions=Index vector (dialog)  Indices=4:6  OutputSizes=1
  Sin : Trigonometry
  Sum : Sum  Inputs=|+-
  Sum1 : Sum  Inputs=|++
  Sum2 : Sum  Inputs=|+-
  Sum3 : Sum  Inputs=|++
  vec2skew : Subsystem
  p : Outport
  wires:
  Product/1 -> Sum1/2
  q/1 -> Cos/1, Product/1, Sin/1, Sum2/1
  Cos/1 -> Sum/2
  Constant/1 -> Sum/1
  vec2skew/1("[x]") -> Matrix Multiply/2, Matrix Multiply/1, Product1/1  "[w]"
  Sum2/1 -> Product2/2
  I/1 -> Product/2
  Product1/1 -> Sum1/1
  Sum/1 -> Product1/2
  Matrix Multiply/1 -> Product2/1  "[v]^2"
  Sum3/1 -> Matrix Multiply1/1
  Product2/1 -> Sum3/2
  Sin/1 -> Sum2/2
  Sum1/1 -> Sum3/1
  Selector1/1 -> Matrix Multiply1/2  "v"
  Matrix Multiply1/1 -> p/1
  Selector/1 -> vec2skew/1(x)  "w"
  S/1 -> Selector1/1, Selector/1

== system rr_arm_control/link_2/spaceJacobian/angle_screw_to_tform/tform ==
  R : Inport
  p : Inport  Port=2
  Constant : Constant  Value=[0,0,0,1]
  Matrix Concatenate : Concatenate  Mode=Multidimensional array  ConcatenateDimension=2
  Matrix Concatenate2 : Concatenate  Mode=Multidimensional array
  Reshape : Reshape  OutputDimensionality=Row vector (2-D)
  T : Outport
  wires:
  p/1 -> Matrix Concatenate/2
  Constant/1 -> Reshape/1
  Matrix Concatenate/1 -> Matrix Concatenate2/1
  Matrix Concatenate2/1 -> T/1
  R/1 -> Matrix Concatenate/1
  Reshape/1 -> Matrix Concatenate2/2

== system rr_arm_control/link_2/spaceJacobian/tform_adjoint/vec2skew ==
  x : Inport
  Constant : Constant  Value=0
  Demux : Demux  Outputs=3
  Gain : Gain  Gain=-1
  Gain1 : Gain  Gain=-1
  Gain2 : Gain  Gain=-1
  Matrix Concatenate : Concatenate  NumInputs=3  Mode=Multidimensional array  ConcatenateDimension=2
  Mux : Mux  Inputs=3
  Mux1 : Mux  Inputs=3
  Mux2 : Mux  Inputs=3
  "[x]" : Outport
  wires:
  Mux1/1 -> Matrix Concatenate/2
  Mux/1 -> Matrix Concatenate/1
  Mux2/1 -> Matrix Concatenate/3
  Matrix Concatenate/1 -> "[x]"/1
  Gain/1 -> Mux/3
  Gain1/1 -> Mux1/1
  Gain2/1 -> Mux2/2
  Constant/1 -> Mux/1, Mux1/2, Mux2/3
  x/1 -> Demux/1
  Demux/3 -> Gain1/1, Mux/2  "z"
  Demux/2 -> Mux2/1, Gain/1  "y"
  Demux/1 -> Gain2/1, Mux1/3  "x"

== system rr_arm_control/link_2/spaceJacobianRate/angle_screw_to_tform/axisAngleToRotMat ==
  w : Inport
  q : Inport  Port=2
  Constant : Constant
  Cos : Trigonometry  Operator=cos
  I : Constant  Value=eye(3)
  Matrix Multiply : Product  Multiplication=Matrix(*)
  Product : Product
  Product1 : Product
  Sin : Trigonometry
  Sum : Sum  Inputs=|+-
  Sum1 : Sum  Inputs=|++
  Sum2 : Sum  Inputs=|++
  vec2skew : Subsystem
  R : Outport
  wires:
  Cos/1 -> Sum/2
  Sum1/1 -> Sum2/1
  Sum/1 -> Product1/2
  Matrix Multiply/1 -> Product1/1  "[w]^2"
  Product1/1 -> Sum1/2
  Constant/1 -> Sum/1
  Product/1 -> Sum1/1
  I/1 -> Sum2/2
  vec2skew/1("[x]") -> Matrix Multiply/2, Matrix Multiply/1, Product/1  "[w]"
  Sin/1 -> Product/2
  q/1 -> Cos/1, Sin/1
  Sum2/1 -> R/1
  w/1 -> vec2skew/1(x)

== system rr_arm_control/link_2/spaceJacobianRate/angle_screw_to_tform/screwDistanceToPos ==
  S : Inport
  q : Inport  Port=2
  Constant : Constant
  Cos : Trigonometry  Operator=cos
  I : Constant  Value=eye(3)
  Matrix Multiply : Product  Multiplication=Matrix(*)
  Matrix Multiply1 : Product  Multiplication=Matrix(*)
  Product : Product
  Product1 : Product
  Product2 : Product
  Selector : Selector  InputPortWidth=6  IndexOptions=Index vector (dialog)  Indices=1:3  OutputSizes=1
  Selector1 : Selector  InputPortWidth=6  IndexOptions=Index vector (dialog)  Indices=4:6  OutputSizes=1
  Sin : Trigonometry
  Sum : Sum  Inputs=|+-
  Sum1 : Sum  Inputs=|++
  Sum2 : Sum  Inputs=|+-
  Sum3 : Sum  Inputs=|++
  vec2skew : Subsystem
  p : Outport
  wires:
  Product/1 -> Sum1/2
  q/1 -> Cos/1, Product/1, Sin/1, Sum2/1
  Cos/1 -> Sum/2
  Constant/1 -> Sum/1
  vec2skew/1("[x]") -> Matrix Multiply/2, Matrix Multiply/1, Product1/1  "[w]"
  Sum2/1 -> Product2/2
  I/1 -> Product/2
  Product1/1 -> Sum1/1
  Sum/1 -> Product1/2
  Matrix Multiply/1 -> Product2/1  "[v]^2"
  Sum3/1 -> Matrix Multiply1/1
  Product2/1 -> Sum3/2
  Sin/1 -> Sum2/2
  Sum1/1 -> Sum3/1
  Selector1/1 -> Matrix Multiply1/2  "v"
  Matrix Multiply1/1 -> p/1
  Selector/1 -> vec2skew/1(x)  "w"
  S/1 -> Selector1/1, Selector/1

== system rr_arm_control/link_2/spaceJacobianRate/angle_screw_to_tform/tform ==
  R : Inport
  p : Inport  Port=2
  Constant : Constant  Value=[0,0,0,1]
  Matrix Concatenate : Concatenate  Mode=Multidimensional array  ConcatenateDimension=2
  Matrix Concatenate2 : Concatenate  Mode=Multidimensional array
  Reshape : Reshape  OutputDimensionality=Row vector (2-D)
  T : Outport
  wires:
  p/1 -> Matrix Concatenate/2
  Constant/1 -> Reshape/1
  Matrix Concatenate/1 -> Matrix Concatenate2/1
  Matrix Concatenate2/1 -> T/1
  R/1 -> Matrix Concatenate/1
  Reshape/1 -> Matrix Concatenate2/2

== system rr_arm_control/link_2/spaceJacobianRate/tform_adjoint/vec2skew ==
  x : Inport
  Constant : Constant  Value=0
  Demux : Demux  Outputs=3
  Gain : Gain  Gain=-1
  Gain1 : Gain  Gain=-1
  Gain2 : Gain  Gain=-1
  Matrix Concatenate : Concatenate  NumInputs=3  Mode=Multidimensional array  ConcatenateDimension=2
  Mux : Mux  Inputs=3
  Mux1 : Mux  Inputs=3
  Mux2 : Mux  Inputs=3
  "[x]" : Outport
  wires:
  Mux1/1 -> Matrix Concatenate/2
  Mux/1 -> Matrix Concatenate/1
  Mux2/1 -> Matrix Concatenate/3
  Matrix Concatenate/1 -> "[x]"/1
  Gain/1 -> Mux/3
  Gain1/1 -> Mux1/1
  Gain2/1 -> Mux2/2
  Constant/1 -> Mux/1, Mux1/2, Mux2/3
  x/1 -> Demux/1
  Demux/3 -> Gain1/1, Mux/2  "z"
  Demux/2 -> Mux2/1, Gain/1  "y"
  Demux/1 -> Gain2/1, Mux1/3  "x"

== system rr_arm_control/link_2/spaceJacobianRate/twist_adjoint/[v] ==
  x : Inport
  Constant : Constant  Value=0
  Demux : Demux  Outputs=3
  Gain : Gain  Gain=-1
  Gain1 : Gain  Gain=-1
  Gain2 : Gain  Gain=-1
  Matrix Concatenate : Concatenate  NumInputs=3  Mode=Multidimensional array  ConcatenateDimension=2
  Mux : Mux  Inputs=3
  Mux1 : Mux  Inputs=3
  Mux2 : Mux  Inputs=3
  "[x]" : Outport
  wires:
  Mux1/1 -> Matrix Concatenate/2
  Mux/1 -> Matrix Concatenate/1
  Mux2/1 -> Matrix Concatenate/3
  Matrix Concatenate/1 -> "[x]"/1
  Gain/1 -> Mux/3
  Gain1/1 -> Mux1/1
  Gain2/1 -> Mux2/2
  Constant/1 -> Mux/1, Mux1/2, Mux2/3
  x/1 -> Demux/1
  Demux/3 -> Gain1/1, Mux/2  "z"
  Demux/2 -> Mux2/1, Gain/1  "y"
  Demux/1 -> Gain2/1, Mux1/3  "x"

== system rr_arm_control/link_2/spaceJacobianRate/twist_adjoint/[w] ==
  x : Inport
  Constant : Constant  Value=0
  Demux : Demux  Outputs=3
  Gain : Gain  Gain=-1
  Gain1 : Gain  Gain=-1
  Gain2 : Gain  Gain=-1
  Matrix Concatenate : Concatenate  NumInputs=3  Mode=Multidimensional array  ConcatenateDimension=2
  Mux : Mux  Inputs=3
  Mux1 : Mux  Inputs=3
  Mux2 : Mux  Inputs=3
  "[x]" : Outport
  wires:
  Mux1/1 -> Matrix Concatenate/2
  Mux/1 -> Matrix Concatenate/1
  Mux2/1 -> Matrix Concatenate/3
  Matrix Concatenate/1 -> "[x]"/1
  Gain/1 -> Mux/3
  Gain1/1 -> Mux1/1
  Gain2/1 -> Mux2/2
  Constant/1 -> Mux/1, Mux1/2, Mux2/3
  x/1 -> Demux/1
  Demux/3 -> Gain1/1, Mux/2  "z"
  Demux/2 -> Mux2/1, Gain/1  "y"
  Demux/1 -> Gain2/1, Mux1/3  "x"

== system rr_arm_control/link_1/productOfExponentials/Subsystem1/axisAngleToRotMat/vec2skew ==
  x : Inport
  Constant : Constant  Value=0
  Demux : Demux  Outputs=3
  Gain : Gain  Gain=-1
  Gain1 : Gain  Gain=-1
  Gain2 : Gain  Gain=-1
  Matrix Concatenate : Concatenate  NumInputs=3  Mode=Multidimensional array  ConcatenateDimension=2
  Mux : Mux  Inputs=3
  Mux1 : Mux  Inputs=3
  Mux2 : Mux  Inputs=3
  "[x]" : Outport
  wires:
  Mux1/1 -> Matrix Concatenate/2
  Mux/1 -> Matrix Concatenate/1
  Mux2/1 -> Matrix Concatenate/3
  Matrix Concatenate/1 -> "[x]"/1
  Gain/1 -> Mux/3
  Gain1/1 -> Mux1/1
  Gain2/1 -> Mux2/2
  Constant/1 -> Mux/1, Mux1/2, Mux2/3
  x/1 -> Demux/1
  Demux/3 -> Gain1/1, Mux/2  "z"
  Demux/2 -> Mux2/1, Gain/1  "y"
  Demux/1 -> Gain2/1, Mux1/3  "x"

== system rr_arm_control/link_1/productOfExponentials/Subsystem1/screwDistanceToPos/vec2skew ==
  x : Inport
  Constant : Constant  Value=0
  Demux : Demux  Outputs=3
  Gain : Gain  Gain=-1
  Gain1 : Gain  Gain=-1
  Gain2 : Gain  Gain=-1
  Matrix Concatenate : Concatenate  NumInputs=3  Mode=Multidimensional array  ConcatenateDimension=2
  Mux : Mux  Inputs=3
  Mux1 : Mux  Inputs=3
  Mux2 : Mux  Inputs=3
  "[x]" : Outport
  wires:
  Mux1/1 -> Matrix Concatenate/2
  Mux/1 -> Matrix Concatenate/1
  Mux2/1 -> Matrix Concatenate/3
  Matrix Concatenate/1 -> "[x]"/1
  Gain/1 -> Mux/3
  Gain1/1 -> Mux1/1
  Gain2/1 -> Mux2/2
  Constant/1 -> Mux/1, Mux1/2, Mux2/3
  x/1 -> Demux/1
  Demux/3 -> Gain1/1, Mux/2  "z"
  Demux/2 -> Mux2/1, Gain/1  "y"
  Demux/1 -> Gain2/1, Mux1/3  "x"

== system rr_arm_control/link_1/spaceJacobian/angle_screw_to_tform/axisAngleToRotMat/vec2skew ==
  x : Inport
  Constant : Constant  Value=0
  Demux : Demux  Outputs=3
  Gain : Gain  Gain=-1
  Gain1 : Gain  Gain=-1
  Gain2 : Gain  Gain=-1
  Matrix Concatenate : Concatenate  NumInputs=3  Mode=Multidimensional array  ConcatenateDimension=2
  Mux : Mux  Inputs=3
  Mux1 : Mux  Inputs=3
  Mux2 : Mux  Inputs=3
  "[x]" : Outport
  wires:
  Mux1/1 -> Matrix Concatenate/2
  Mux/1 -> Matrix Concatenate/1
  Mux2/1 -> Matrix Concatenate/3
  Matrix Concatenate/1 -> "[x]"/1
  Gain/1 -> Mux/3
  Gain1/1 -> Mux1/1
  Gain2/1 -> Mux2/2
  Constant/1 -> Mux/1, Mux1/2, Mux2/3
  x/1 -> Demux/1
  Demux/3 -> Gain1/1, Mux/2  "z"
  Demux/2 -> Mux2/1, Gain/1  "y"
  Demux/1 -> Gain2/1, Mux1/3  "x"

== system rr_arm_control/link_1/spaceJacobian/angle_screw_to_tform/screwDistanceToPos/vec2skew ==
  x : Inport
  Constant : Constant  Value=0
  Demux : Demux  Outputs=3
  Gain : Gain  Gain=-1
  Gain1 : Gain  Gain=-1
  Gain2 : Gain  Gain=-1
  Matrix Concatenate : Concatenate  NumInputs=3  Mode=Multidimensional array  ConcatenateDimension=2
  Mux : Mux  Inputs=3
  Mux1 : Mux  Inputs=3
  Mux2 : Mux  Inputs=3
  "[x]" : Outport
  wires:
  Mux1/1 -> Matrix Concatenate/2
  Mux/1 -> Matrix Concatenate/1
  Mux2/1 -> Matrix Concatenate/3
  Matrix Concatenate/1 -> "[x]"/1
  Gain/1 -> Mux/3
  Gain1/1 -> Mux1/1
  Gain2/1 -> Mux2/2
  Constant/1 -> Mux/1, Mux1/2, Mux2/3
  x/1 -> Demux/1
  Demux/3 -> Gain1/1, Mux/2  "z"
  Demux/2 -> Mux2/1, Gain/1  "y"
  Demux/1 -> Gain2/1, Mux1/3  "x"

== system rr_arm_control/link_1/spaceJacobianRate/angle_screw_to_tform/axisAngleToRotMat/vec2skew ==
  x : Inport
  Constant : Constant  Value=0
  Demux : Demux  Outputs=3
  Gain : Gain  Gain=-1
  Gain1 : Gain  Gain=-1
  Gain2 : Gain  Gain=-1
  Matrix Concatenate : Concatenate  NumInputs=3  Mode=Multidimensional array  ConcatenateDimension=2
  Mux : Mux  Inputs=3
  Mux1 : Mux  Inputs=3
  Mux2 : Mux  Inputs=3
  "[x]" : Outport
  wires:
  Mux1/1 -> Matrix Concatenate/2
  Mux/1 -> Matrix Concatenate/1
  Mux2/1 -> Matrix Concatenate/3
  Matrix Concatenate/1 -> "[x]"/1
  Gain/1 -> Mux/3
  Gain1/1 -> Mux1/1
  Gain2/1 -> Mux2/2
  Constant/1 -> Mux/1, Mux1/2, Mux2/3
  x/1 -> Demux/1
  Demux/3 -> Gain1/1, Mux/2  "z"
  Demux/2 -> Mux2/1, Gain/1  "y"
  Demux/1 -> Gain2/1, Mux1/3  "x"

== system rr_arm_control/link_1/spaceJacobianRate/angle_screw_to_tform/screwDistanceToPos/vec2skew ==
  x : Inport
  Constant : Constant  Value=0
  Demux : Demux  Outputs=3
  Gain : Gain  Gain=-1
  Gain1 : Gain  Gain=-1
  Gain2 : Gain  Gain=-1
  Matrix Concatenate : Concatenate  NumInputs=3  Mode=Multidimensional array  ConcatenateDimension=2
  Mux : Mux  Inputs=3
  Mux1 : Mux  Inputs=3
  Mux2 : Mux  Inputs=3
  "[x]" : Outport
  wires:
  Mux1/1 -> Matrix Concatenate/2
  Mux/1 -> Matrix Concatenate/1
  Mux2/1 -> Matrix Concatenate/3
  Matrix Concatenate/1 -> "[x]"/1
  Gain/1 -> Mux/3
  Gain1/1 -> Mux1/1
  Gain2/1 -> Mux2/2
  Constant/1 -> Mux/1, Mux1/2, Mux2/3
  x/1 -> Demux/1
  Demux/3 -> Gain1/1, Mux/2  "z"
  Demux/2 -> Mux2/1, Gain/1  "y"
  Demux/1 -> Gain2/1, Mux1/3  "x"

== system rr_arm_control/link_2/productOfExponentials/Subsystem1/axisAngleToRotMat/vec2skew ==
  x : Inport
  Constant : Constant  Value=0
  Demux : Demux  Outputs=3
  Gain : Gain  Gain=-1
  Gain1 : Gain  Gain=-1
  Gain2 : Gain  Gain=-1
  Matrix Concatenate : Concatenate  NumInputs=3  Mode=Multidimensional array  ConcatenateDimension=2
  Mux : Mux  Inputs=3
  Mux1 : Mux  Inputs=3
  Mux2 : Mux  Inputs=3
  "[x]" : Outport
  wires:
  Mux1/1 -> Matrix Concatenate/2
  Mux/1 -> Matrix Concatenate/1
  Mux2/1 -> Matrix Concatenate/3
  Matrix Concatenate/1 -> "[x]"/1
  Gain/1 -> Mux/3
  Gain1/1 -> Mux1/1
  Gain2/1 -> Mux2/2
  Constant/1 -> Mux/1, Mux1/2, Mux2/3
  x/1 -> Demux/1
  Demux/3 -> Gain1/1, Mux/2  "z"
  Demux/2 -> Mux2/1, Gain/1  "y"
  Demux/1 -> Gain2/1, Mux1/3  "x"

== system rr_arm_control/link_2/productOfExponentials/Subsystem1/screwDistanceToPos/vec2skew ==
  x : Inport
  Constant : Constant  Value=0
  Demux : Demux  Outputs=3
  Gain : Gain  Gain=-1
  Gain1 : Gain  Gain=-1
  Gain2 : Gain  Gain=-1
  Matrix Concatenate : Concatenate  NumInputs=3  Mode=Multidimensional array  ConcatenateDimension=2
  Mux : Mux  Inputs=3
  Mux1 : Mux  Inputs=3
  Mux2 : Mux  Inputs=3
  "[x]" : Outport
  wires:
  Mux1/1 -> Matrix Concatenate/2
  Mux/1 -> Matrix Concatenate/1
  Mux2/1 -> Matrix Concatenate/3
  Matrix Concatenate/1 -> "[x]"/1
  Gain/1 -> Mux/3
  Gain1/1 -> Mux1/1
  Gain2/1 -> Mux2/2
  Constant/1 -> Mux/1, Mux1/2, Mux2/3
  x/1 -> Demux/1
  Demux/3 -> Gain1/1, Mux/2  "z"
  Demux/2 -> Mux2/1, Gain/1  "y"
  Demux/1 -> Gain2/1, Mux1/3  "x"

== system rr_arm_control/link_2/spaceJacobian/angle_screw_to_tform/axisAngleToRotMat/vec2skew ==
  x : Inport
  Constant : Constant  Value=0
  Demux : Demux  Outputs=3
  Gain : Gain  Gain=-1
  Gain1 : Gain  Gain=-1
  Gain2 : Gain  Gain=-1
  Matrix Concatenate : Concatenate  NumInputs=3  Mode=Multidimensional array  ConcatenateDimension=2
  Mux : Mux  Inputs=3
  Mux1 : Mux  Inputs=3
  Mux2 : Mux  Inputs=3
  "[x]" : Outport
  wires:
  Mux1/1 -> Matrix Concatenate/2
  Mux/1 -> Matrix Concatenate/1
  Mux2/1 -> Matrix Concatenate/3
  Matrix Concatenate/1 -> "[x]"/1
  Gain/1 -> Mux/3
  Gain1/1 -> Mux1/1
  Gain2/1 -> Mux2/2
  Constant/1 -> Mux/1, Mux1/2, Mux2/3
  x/1 -> Demux/1
  Demux/3 -> Gain1/1, Mux/2  "z"
  Demux/2 -> Mux2/1, Gain/1  "y"
  Demux/1 -> Gain2/1, Mux1/3  "x"

== system rr_arm_control/link_2/spaceJacobian/angle_screw_to_tform/screwDistanceToPos/vec2skew ==
  x : Inport
  Constant : Constant  Value=0
  Demux : Demux  Outputs=3
  Gain : Gain  Gain=-1
  Gain1 : Gain  Gain=-1
  Gain2 : Gain  Gain=-1
  Matrix Concatenate : Concatenate  NumInputs=3  Mode=Multidimensional array  ConcatenateDimension=2
  Mux : Mux  Inputs=3
  Mux1 : Mux  Inputs=3
  Mux2 : Mux  Inputs=3
  "[x]" : Outport
  wires:
  Mux1/1 -> Matrix Concatenate/2
  Mux/1 -> Matrix Concatenate/1
  Mux2/1 -> Matrix Concatenate/3
  Matrix Concatenate/1 -> "[x]"/1
  Gain/1 -> Mux/3
  Gain1/1 -> Mux1/1
  Gain2/1 -> Mux2/2
  Constant/1 -> Mux/1, Mux1/2, Mux2/3
  x/1 -> Demux/1
  Demux/3 -> Gain1/1, Mux/2  "z"
  Demux/2 -> Mux2/1, Gain/1  "y"
  Demux/1 -> Gain2/1, Mux1/3  "x"

== system rr_arm_control/link_2/spaceJacobianRate/angle_screw_to_tform/axisAngleToRotMat/vec2skew ==
  x : Inport
  Constant : Constant  Value=0
  Demux : Demux  Outputs=3
  Gain : Gain  Gain=-1
  Gain1 : Gain  Gain=-1
  Gain2 : Gain  Gain=-1
  Matrix Concatenate : Concatenate  NumInputs=3  Mode=Multidimensional array  ConcatenateDimension=2
  Mux : Mux  Inputs=3
  Mux1 : Mux  Inputs=3
  Mux2 : Mux  Inputs=3
  "[x]" : Outport
  wires:
  Mux1/1 -> Matrix Concatenate/2
  Mux/1 -> Matrix Concatenate/1
  Mux2/1 -> Matrix Concatenate/3
  Matrix Concatenate/1 -> "[x]"/1
  Gain/1 -> Mux/3
  Gain1/1 -> Mux1/1
  Gain2/1 -> Mux2/2
  Constant/1 -> Mux/1, Mux1/2, Mux2/3
  x/1 -> Demux/1
  Demux/3 -> Gain1/1, Mux/2  "z"
  Demux/2 -> Mux2/1, Gain/1  "y"
  Demux/1 -> Gain2/1, Mux1/3  "x"

== system rr_arm_control/link_2/spaceJacobianRate/angle_screw_to_tform/screwDistanceToPos/vec2skew ==
  x : Inport
  Constant : Constant  Value=0
  Demux : Demux  Outputs=3
  Gain : Gain  Gain=-1
  Gain1 : Gain  Gain=-1
  Gain2 : Gain  Gain=-1
  Matrix Concatenate : Concatenate  NumInputs=3  Mode=Multidimensional array  ConcatenateDimension=2
  Mux : Mux  Inputs=3
  Mux1 : Mux  Inputs=3
  Mux2 : Mux  Inputs=3
  "[x]" : Outport
  wires:
  Mux1/1 -> Matrix Concatenate/2
  Mux/1 -> Matrix Concatenate/1
  Mux2/1 -> Matrix Concatenate/3
  Matrix Concatenate/1 -> "[x]"/1
  Gain/1 -> Mux/3
  Gain1/1 -> Mux1/1
  Gain2/1 -> Mux2/2
  Constant/1 -> Mux/1, Mux1/2, Mux2/3
  x/1 -> Demux/1
  Demux/3 -> Gain1/1, Mux/2  "z"
  Demux/2 -> Mux2/1, Gain/1  "y"
  Demux/1 -> Gain2/1, Mux1/3  "x"

== matlab function rr_arm_control/MATLAB Function ==
  data: q input size=[2,1]; dq input size=[2,1]; ddq output size=[4,1]; params input
function ddq = fcn(q,dq,params)
M = rrarmMassMatrix([q;dq],zeros(2,1),params);
f = rrarmForcingVector([q;dq],zeros(2,1),params);
ddq = M\f;
